simulink model "interbotix"  (R2024a)
settings: Solver=VariableStepAuto  StartTime=0.0  StopTime=10.0  RelTol=1e-3
libraries: ros2lib x7
settings Model: Creator=deivideich  LastModifiedBy=deivideich

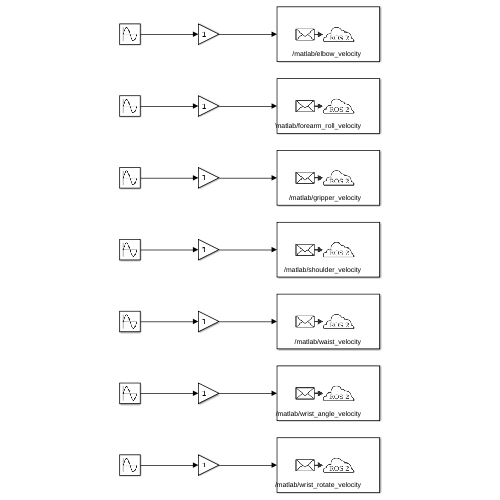
[thumbnail: Simulink's stored preview of the top-level diagram]
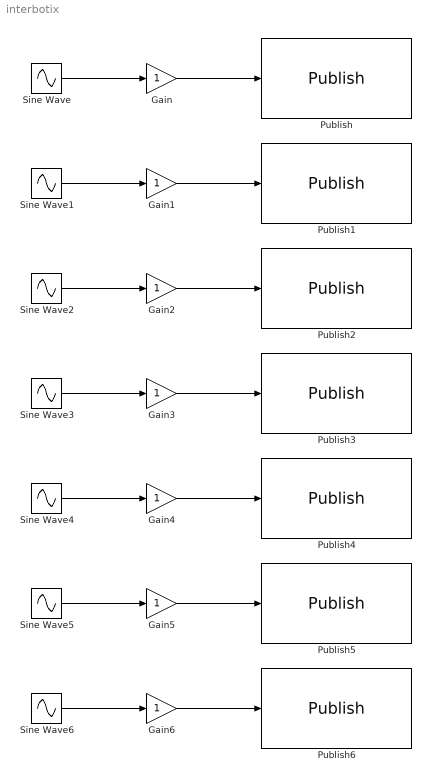
== system interbotix ==
  Gain{,1..6} (7 alike) : Gain
  Publish : ros2lib/Publish  topicSource=Select from ROS network  topic=/matlab/elbow_velocity  messageType=std_msgs/Float32  QOSHistory=Keep last  QOSDepth=1  QOSReliability=Reliable  QOSDurability=Volatile  QOSDeadline=Inf  QOSLifespan=Inf  QOSLiveliness=Automatic  QOSLeaseDuration=Inf  QOSAvoidROSNamespaceConventions=off
  Publish1 : ros2lib/Publish  topicSource=Select from ROS network  topic=/matlab/forearm_roll_velocity  messageType=std_msgs/Float32  QOSHistory=Keep last  QOSDepth=1  QOSReliability=Reliable  QOSDurability=Volatile  QOSDeadline=Inf  QOSLifespan=Inf  QOSLiveliness=Automatic  QOSLeaseDuration=Inf  QOSAvoidROSNamespaceConventions=off
  Publish2 : ros2lib/Publish  topicSource=Select from ROS network  topic=/matlab/gripper_velocity  messageType=std_msgs/Float32  QOSHistory=Keep last  QOSDepth=1  QOSReliability=Reliable  QOSDurability=Volatile  QOSDeadline=Inf  QOSLifespan=Inf  QOSLiveliness=Automatic  QOSLeaseDuration=Inf  QOSAvoidROSNamespaceConventions=off
  Publish3 : ros2lib/Publish  topicSource=Select from ROS network  topic=/matlab/shoulder_velocity  messageType=std_msgs/Float32  QOSHistory=Keep last  QOSDepth=1  QOSReliability=Reliable  QOSDurability=Volatile  QOSDeadline=Inf  QOSLifespan=Inf  QOSLiveliness=Automatic  QOSLeaseDuration=Inf  QOSAvoidROSNamespaceConventions=off
  Publish4 : ros2lib/Publish  topicSource=Select from ROS network  topic=/matlab/waist_velocity  messageType=std_msgs/Float32  QOSHistory=Keep last  QOSDepth=1  QOSReliability=Reliable  QOSDurability=Volatile  QOSDeadline=Inf  QOSLifespan=Inf  QOSLiveliness=Automatic  QOSLeaseDuration=Inf  QOSAvoidROSNamespaceConventions=off
  Publish5 : ros2lib/Publish  topicSource=Select from ROS network  topic=/matlab/wrist_angle_velocity  messageType=std_msgs/Float32  QOSHistory=Keep last  QOSDepth=1  QOSReliability=Reliable  QOSDurability=Volatile  QOSDeadline=Inf  QOSLifespan=Inf  QOSLiveliness=Automatic  QOSLeaseDuration=Inf  QOSAvoidROSNamespaceConventions=off
  Publish6 : ros2lib/Publish  topicSource=Select from ROS network  topic=/matlab/wrist_rotate_velocity  messageType=std_msgs/Float32  QOSHistory=Keep last  QOSDepth=1  QOSReliability=Reliable  QOSDurability=Volatile  QOSDeadline=Inf  QOSLifespan=Inf  QOSLiveliness=Automatic  QOSLeaseDuration=Inf  QOSAvoidROSNamespaceConventions=off
  Sine Wave{,1..6} (7 alike) : Sin  SampleTime=0
  wires:
  Sine Wave/1 -> Gain/1
  Gain/1 -> Publish/1
  Sine Wave1/1 -> Gain1/1
  Gain1/1 -> Publish1/1
  Sine Wave3/1 -> Gain3/1
  Sine Wave2/1 -> Gain2/1
  Gain3/1 -> Publish3/1
  Gain2/1 -> Publish2/1
  Sine Wave5/1 -> Gain5/1
  Sine Wave4/1 -> Gain4/1
  Gain5/1 -> Publish5/1
  Gain4/1 -> Publish4/1
  Sine Wave6/1 -> Gain6/1
  Gain6/1 -> Publish6/1
